simulink model "simulink_trot_discret"  (R2023a)
settings: Solver=VariableStepAuto  StartTime=0.0  StopTime=10  RelTol=1e-3
values from neighbouring files (symbols this model uses):
  denum_filtre = denum_ordre1    [Script_BE.m]
  Gain_Capteur = Gain_LEM    (= 0.104)    [Script_BE.m]
  K_Corr = K_LEM    (= 0.503460361152)    [Script_BE.m]
  L = 2*10^-3    (= 0.002)    [Script_BE.m]
  num_filtre = num_ordre1    [Script_BE.m]
  tau_i = tau_i_lem    (= 0.00397250737957)    [Script_BE.m]
  Te = 1/Fe    (= 0.0005)    [Script_BE.m]
  U_bat = 24    [Script_BE.m]
settings Model: Creator=bogen  LastModifiedBy=bogen

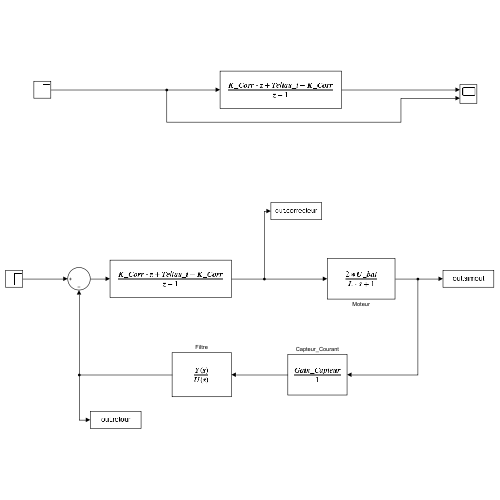
[thumbnail: Simulink's stored preview of the top-level diagram]
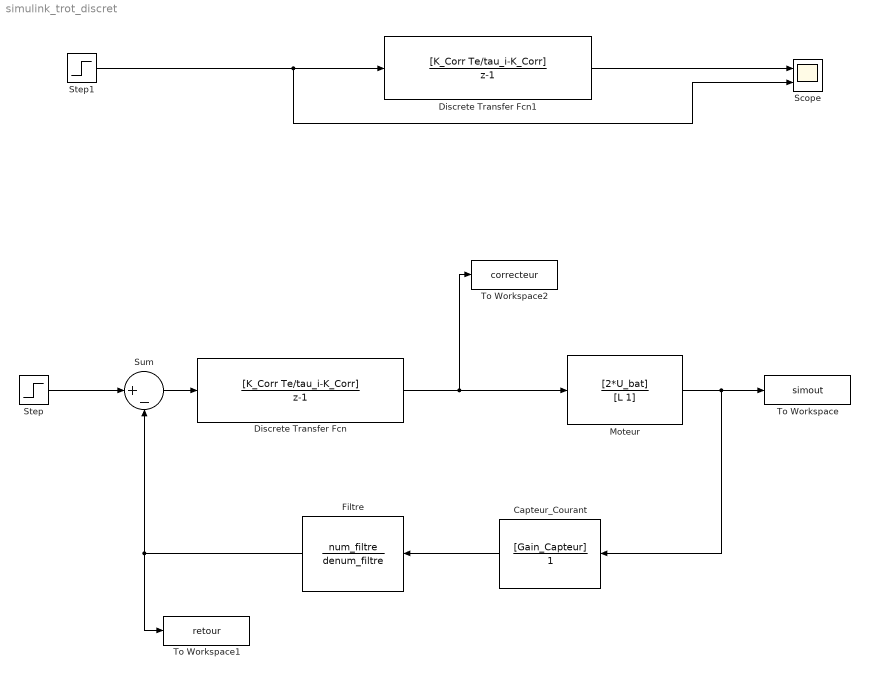
== system simulink_trot_discret ==
  Capteur_Courant : TransferFcn  Numerator=[Gain_Capteur]  Denominator=[1]
  Discrete Transfer Fcn : DiscreteTransferFcn  Numerator=[K_Corr Te/tau_i-K_Corr]  Denominator=[1 -1]  SampleTime=Te
  Discrete Transfer Fcn1 : DiscreteTransferFcn  Numerator=[K_Corr Te/tau_i-K_Corr]  Denominator=[1 -1]  SampleTime=Te
  Filtre : TransferFcn  Numerator=num_filtre  Denominator=denum_filtre
  Moteur : TransferFcn  Numerator=[2*U_bat]  Denominator=[L 1]
  Scope : Scope  NumInputPorts=2
  Step : Step  After=3.3  SampleTime=0
  Step1 : Step  After=0.2  SampleTime=Te
  Sum : Sum  Inputs=|+-
  To Workspace : ToWorkspace  VariableName=simout  SaveFormat=Timeseries  SampleTime=-1
  To Workspace1 : ToWorkspace  VariableName=retour  SaveFormat=Timeseries  SampleTime=-1
  To Workspace2 : ToWorkspace  VariableName=correcteur  SaveFormat=Timeseries  SampleTime=-1
  wires:
  Discrete Transfer Fcn/1 -> To Workspace2/1, Moteur/1
  Moteur/1 -> Capteur_Courant/1, To Workspace/1
  Capteur_Courant/1 -> Filtre/1
  Filtre/1 -> To Workspace1/1, Sum/2
  Step/1 -> Sum/1
  Sum/1 -> Discrete Transfer Fcn/1
  Step1/1 -> Scope/2, Discrete Transfer Fcn1/1
  Discrete Transfer Fcn1/1 -> Scope/1
